simulink library "lib_moving_average_filter"  (R2023a)
settings: Solver=VariableStepAuto  StartTime=0.0  StopTime=10.0  RelTol=1e-3
libraries: simulink x1, lib_conversion x1
settings Model: Creator=cav2ofo  LastModifiedBy=xiaoqiang.yuan
settings OptimizationCC: ReuseModelBlockBuffer=off

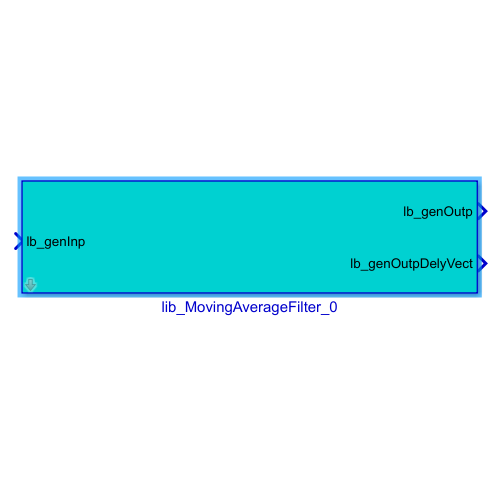
[thumbnail: Simulink's stored preview of the top-level diagram]
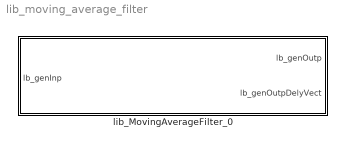
== system lib_moving_average_filter ==
  lib_MovingAverageFilter_0 : Subsystem  mask{lb_parSampNum=10, lb_parInpSmtnDataType=fixdt(1,32,2^-19,0)}
      mask prompts: lb_parSampNum "Samplings number:"; lb_parInpSmtnDataType "Input summation data type:"
      mask DialogControl DescGroupVar Prompt: WEIFU motor control library
      mask DialogControl DescTextVar Prompt: Moving average filter
      mask DialogControl Container3 Prompt: Data type:

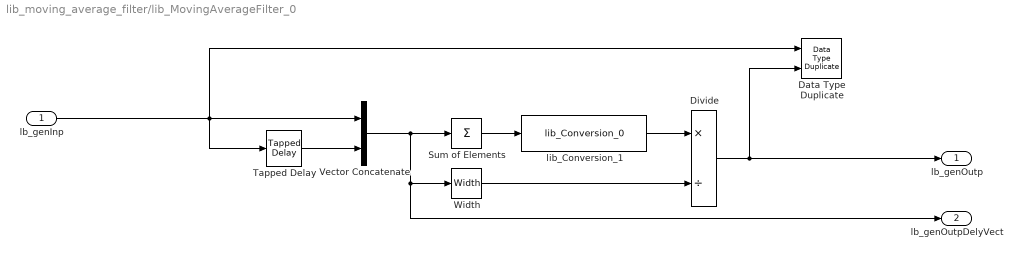
== system lib_moving_average_filter/lib_MovingAverageFilter_0 ==
  "lb_genInp " : Inport
  Data Type Duplicate : DataTypeDuplicate
  Divide : Product  Inputs=*/  OutDataTypeStr=Inherit: Inherit via back propagation  RndMeth=Simplest
  Sum of Elements : Sum  Inputs=+  OutDataTypeStr=Inherit: Inherit via back propagation  RndMeth=Simplest
  Tapped Delay : simulink/Discrete/Tapped Delay  vinit=0  samptime=-1  NumDelays=lb_parSampNum-1  DelayOrder=Oldest  includeCurrent=off
  Vector Concatenate : Concatenate
  Width : Width  DataType=uint16
  lib_Conversion_1 : lib_conversion/lib_Conversion_0  lb_parDataType=lb_parInpSmtnDataType  lb_parOutpMaxVal=[]  lb_parOutpMinVal=[]  lb_parSatFlag=off
  lb_genOutp : Outport  VectorParamsAs1DForOutWhenUnconnected=off
  lb_genOutpDelyVect : Outport  Port=2
  wires:
  "lb_genInp "/1 -> Data Type Duplicate/1, Vector Concatenate/1, Tapped Delay/1
  Tapped Delay/1 -> Vector Concatenate/2
  Sum of Elements/1 -> lib_Conversion_1/1
  Width/1 -> Divide/2
  Divide/1 -> Data Type Duplicate/2, lb_genOutp/1
  lib_Conversion_1/1 -> Divide/1
  Vector Concatenate/1 -> lb_genOutpDelyVect/1, Width/1, Sum of Elements/1
